simulink model "brakeModel"  (R2013b)
settings: Solver=ode3  StartTime=0.0  StopTime=10.0  FixedStep=0.0001  MaxStep=0.01  RelTol=1e-3
InitFcn:
  | initBrakeParams
StartFcn:
  | initBrakeParams
values from neighbouring files (symbols this model uses):
  BF = 0.0001408    [abssim1.mat]    (also in abssim2.mat; abssim3.mat; initBrakeParams.m)
  J = 0.0009    [abssim1.mat]    (also in abssim2.mat; abssim3.mat; espSim1.mat = 0.5; espSim2.mat = 0.5)
  Rd = 0.0625    [abssim1.mat]    (also in abssim2.mat; abssim3.mat; initAbsSim.m)
  v0 = 20    [abssim1.mat]    (also in abssim2.mat; abssim3.mat; initAbsSim.m = 5)
settings Model: FPTRunName=FPA_Reference  Creator=lasse  LastModifiedBy=Lasse
settings OptimizationCC: InlineParams=on
settings DebuggingCC: SignalRangeChecking=warning
settings HardwareCC: ProdBitPerInt=16  ProdBitPerPointer=8  ProdIntDivRoundTo=Zero  ProdEndianess=LittleEndian  ProdWordSize=8  ProdHWDeviceType=Atmel->AVR
settings ModelReferenceCC: ModelReferenceMinAlgLoopOccurrences=on

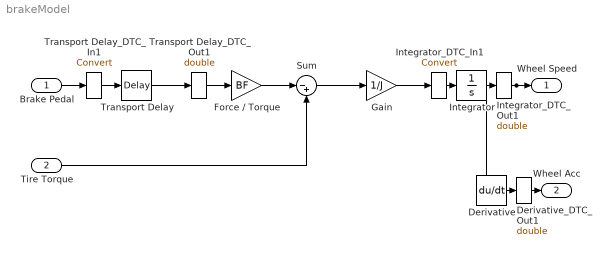
== system brakeModel ==
  Brake Pedal : Inport  OutDataTypeStr=double
  Tire Torque : Inport  Port=2  OutDataTypeStr=double
  Derivative : Derivative
  Derivative_DTC_Out1 : DataTypeConversion  OutDataTypeStr=double
  Force / Torque : Gain  Gain=BF  OutDataTypeStr=double
  Gain : Gain  Gain=1/J  OutDataTypeStr=double
  Integrator : Integrator  InitialCondition=v0/(2*pi*Rd)  LimitOutput=on  LowerSaturationLimit=0
  Integrator_DTC_In1 : DataTypeConversion  LockScale=on
  Integrator_DTC_Out1 : DataTypeConversion  OutDataTypeStr=double  LockScale=on
  Sum : Sum  Inputs=|-+  AccumDataTypeStr=double  OutDataTypeStr=double
  Transport Delay : TransportDelay  DelayTime=0.1
  Transport Delay_DTC_In1 : DataTypeConversion  LockScale=on
  Transport Delay_DTC_Out1 : DataTypeConversion  OutDataTypeStr=double
  Wheel Speed : Outport  OutDataTypeStr=double
  Wheel Acc : Outport  Port=2  OutDataTypeStr=double
  wires:
  Brake Pedal/1 -> Transport Delay_DTC_In1/1
  Force / Torque/1 -> Sum/1
  Tire Torque/1 -> Sum/2
  Sum/1 -> Gain/1
  Gain/1 -> Integrator_DTC_In1/1
  Integrator/1 -> Integrator_DTC_Out1/1
  Transport Delay/1 -> Transport Delay_DTC_Out1/1
  Derivative/1 -> Derivative_DTC_Out1/1
  Transport Delay_DTC_In1/1 -> Transport Delay/1
  Transport Delay_DTC_Out1/1 -> Force / Torque/1
  Integrator_DTC_In1/1 -> Integrator/1
  Integrator_DTC_Out1/1 -> Wheel Speed/1, Derivative/1
  Derivative_DTC_Out1/1 -> Wheel Acc/1
